simulink subsystem "HallSensor"  (R2023a)
settings: Solver=VariableStepAuto  StartTime=0.0  StopTime=10.0  RelTol=1e-3
settings Model: Creator=ycheb  LastModifiedBy=ycheb

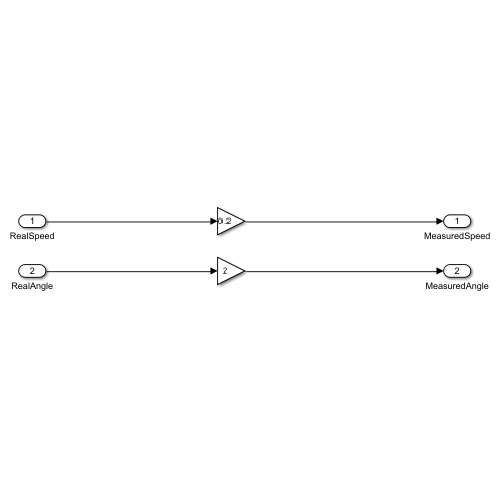
[thumbnail: Simulink's stored preview of the top-level diagram]
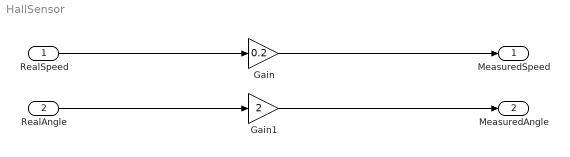
== system HallSensor ==
  RealSpeed : Inport
  RealAngle : Inport  Port=2
  Gain : Gain  Gain=0.2
  Gain1 : Gain  Gain=2
  MeasuredSpeed : Outport
  MeasuredAngle : Outport  Port=2
  wires:
  RealSpeed/1 -> Gain/1
  Gain/1 -> MeasuredSpeed/1
  RealAngle/1 -> Gain1/1
  Gain1/1 -> MeasuredAngle/1
